simulink model "pdeModel"  (R2019a)
settings: Solver=VariableStepAuto  StartTime=0.0  StopTime=20  RelTol=1e-3
settings Model: Creator=wangh  LastModifiedBy=wangh

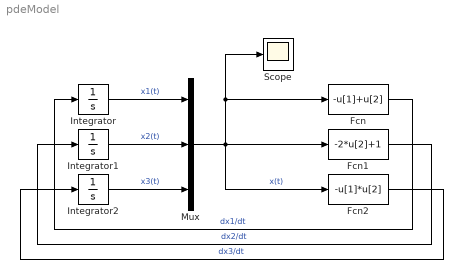
== system pdeModel ==
  Fcn : Fcn  Expr=-u[1]+u[2]
  Fcn1 : Fcn  Expr=-2*u[2]+1
  Fcn2 : Fcn  Expr=-u[1]*u[2]
  Integrator : Integrator  InitialCondition=1
  Integrator1 : Integrator  InitialCondition=1
  Integrator2 : Integrator  InitialCondition=1
  Mux : Mux  Inputs=3
  Scope : Scope
  wires:
  Integrator/1 -> Mux/1  "x1(t)"
  Integrator1/1 -> Mux/2  "x2(t)"
  Integrator2/1 -> Mux/3  "x3(t)"
  Mux/1 -> Fcn2/1, Fcn1/1, Scope/1, Fcn/1  "x(t)"
  Fcn/1 -> Integrator/1  "dx1/dt"
  Fcn1/1 -> Integrator1/1  "dx2/dt"
  Fcn2/1 -> Integrator2/1  "dx3/dt"
